simulink model "mdl_quadrotorLin_16b"  (R2016b)
settings: Solver=ode4  StartTime=0.0  StopTime=20  FixedStep=0.0001  RelTol=1e-3
undefined symbols (not defined in the file or in its folder): Ag_phi_rad, Ag_psi_rad, Ag_theta_rad, AgVel_p_radPerScnd, AgVel_q_radPerScnd, AgVel_r_radPerScnd, par_mdlQuad, par_mdlQuadLin, Pos_z_mtr, V_w_mtrPerScnd
settings Model: Creator=Nu  LastModifiedBy=Nu

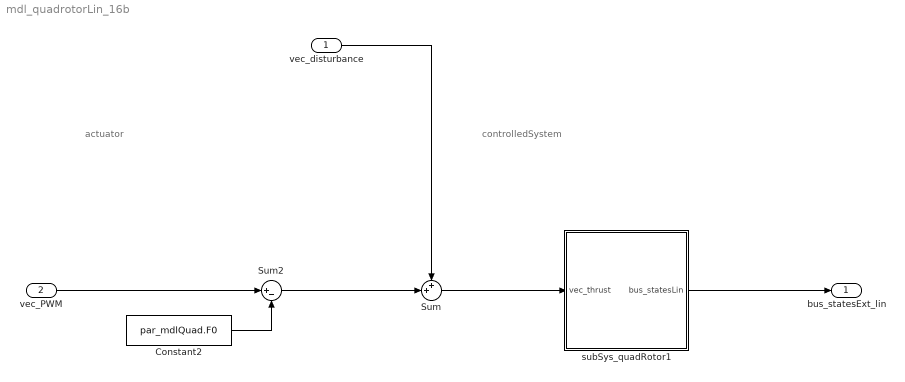
== system mdl_quadrotorLin_16b ==
  note: controlledSystem
  note: actuator
  vec_disturbance : Inport  PortDimensions=4
  vec_PWM : Inport  Port=2  PortDimensions=4
  Constant2 : Constant  Value=par_mdlQuad.F0
  Sum : Sum  Inputs=++|
  Sum2 : Sum  Inputs=|+-
  subSys_quadRotor1 : Subsystem
  bus_statesExt_lin : Outport  OutDataTypeStr=Bus: mdl_statesExt
  wires:
  vec_PWM/1 -> Sum2/1
  vec_disturbance/1 -> Sum/1
  subSys_quadRotor1/1(bus_statesLin) -> bus_statesExt_lin/1
  Constant2/1 -> Sum2/2
  Sum2/1 -> Sum/2
  Sum/1 -> subSys_quadRotor1/1(vec_thrust)

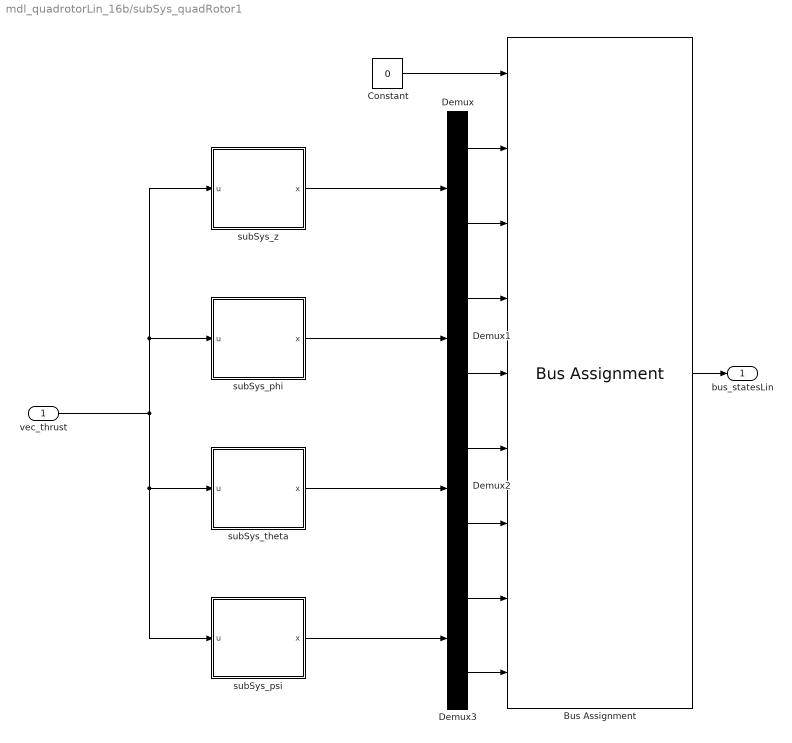
== system mdl_quadrotorLin_16b/subSys_quadRotor1 ==
  vec_thrust : Inport
  Bus Assignment : BusAssignment  AssignedSignals=Pos_z_mtr,V_w_mtrPerScnd,Ag_phi_rad,AgVel_p_radPerScnd,Ag_theta_rad,AgVel_q_radPerScnd,Ag_psi_rad,AgVel_r_radPerScnd
  Constant : Constant  Value=0  OutDataTypeStr=Bus: mdl_statesExt
  Demux{,1..3} (4 alike) : Demux  Outputs=2
  subSys_phi : Subsystem
  subSys_psi : Subsystem
  subSys_theta : Subsystem
  subSys_z : Subsystem
  bus_statesLin : Outport
  wires:
  vec_thrust/1 -> subSys_psi/1(u), subSys_theta/1(u), subSys_phi/1(u), subSys_z/1(u)
  Bus Assignment/1 -> bus_statesLin/1
  Constant/1 -> Bus Assignment/1
  Demux/1 -> Bus Assignment/2
  Demux/2 -> Bus Assignment/3
  Demux1/1 -> Bus Assignment/4
  Demux1/2 -> Bus Assignment/5
  Demux2/1 -> Bus Assignment/6
  Demux2/2 -> Bus Assignment/7
  Demux3/1 -> Bus Assignment/8
  Demux3/2 -> Bus Assignment/9
  subSys_theta/1(x) -> Demux2/1
  subSys_psi/1(x) -> Demux3/1
  subSys_z/1(x) -> Demux/1
  subSys_phi/1(x) -> Demux1/1

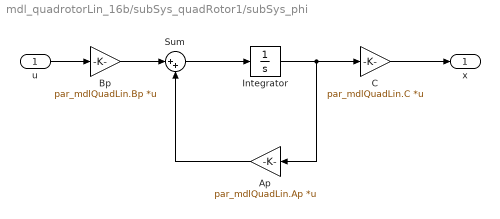
== system mdl_quadrotorLin_16b/subSys_quadRotor1/subSys_phi ==
  u : Inport
  Ap : Gain  Gain=par_mdlQuadLin.Ap  Multiplication=Matrix(K*u)
  Bp : Gain  Gain=par_mdlQuadLin.Bp  Multiplication=Matrix(K*u)
  C : Gain  Gain=par_mdlQuadLin.C  Multiplication=Matrix(K*u)
  Integrator : Integrator
  Sum : Sum  Inputs=|++
  x : Outport
  wires:
  Ap/1 -> Sum/2
  C/1 -> x/1
  Integrator/1 -> C/1, Ap/1
  Sum/1 -> Integrator/1
  Bp/1 -> Sum/1
  u/1 -> Bp/1

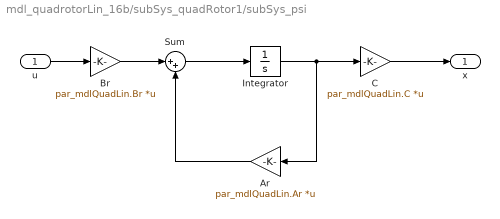
== system mdl_quadrotorLin_16b/subSys_quadRotor1/subSys_psi ==
  u : Inport
  Ar : Gain  Gain=par_mdlQuadLin.Ar  Multiplication=Matrix(K*u)
  Br : Gain  Gain=par_mdlQuadLin.Br  Multiplication=Matrix(K*u)
  C : Gain  Gain=par_mdlQuadLin.C  Multiplication=Matrix(K*u)
  Integrator : Integrator
  Sum : Sum  Inputs=|++
  x : Outport
  wires:
  Ar/1 -> Sum/2
  C/1 -> x/1
  Integrator/1 -> C/1, Ar/1
  Sum/1 -> Integrator/1
  Br/1 -> Sum/1
  u/1 -> Br/1

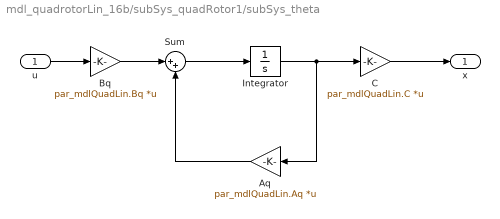
== system mdl_quadrotorLin_16b/subSys_quadRotor1/subSys_theta ==
  u : Inport
  Aq : Gain  Gain=par_mdlQuadLin.Aq  Multiplication=Matrix(K*u)
  Bq : Gain  Gain=par_mdlQuadLin.Bq  Multiplication=Matrix(K*u)
  C : Gain  Gain=par_mdlQuadLin.C  Multiplication=Matrix(K*u)
  Integrator : Integrator
  Sum : Sum  Inputs=|++
  x : Outport
  wires:
  u/1 -> Bq/1
  Bq/1 -> Sum/1
  Sum/1 -> Integrator/1
  Integrator/1 -> Aq/1, C/1
  C/1 -> x/1
  Aq/1 -> Sum/2

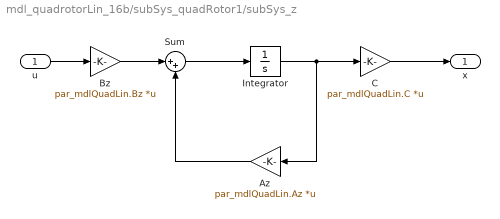
== system mdl_quadrotorLin_16b/subSys_quadRotor1/subSys_z ==
  u : Inport
  Az : Gain  Gain=par_mdlQuadLin.Az  Multiplication=Matrix(K*u)
  Bz : Gain  Gain=par_mdlQuadLin.Bz  Multiplication=Matrix(K*u)
  C : Gain  Gain=par_mdlQuadLin.C  Multiplication=Matrix(K*u)
  Integrator : Integrator
  Sum : Sum  Inputs=|++
  x : Outport
  wires:
  u/1 -> Bz/1
  Bz/1 -> Sum/1
  Sum/1 -> Integrator/1
  Integrator/1 -> Az/1, C/1
  C/1 -> x/1
  Az/1 -> Sum/2
